simulink model "platoon_project"  (Simulink 8.9)
settings: Solver=FixedStepAuto  StartTime=0.0  StopTime=5  FixedStep=0.1  RelTol=1e-3  EnableMultiTasking=on
values from neighbouring files (symbols this model uses):
  tnet_table = [57.5127074443 119.897368421 182.282029398 223.675296349 261.549751738 274.206057597 279.305263158 283.689473684 288.073684211 292.467532318 296.875779086 301.284025854 ... (400 elements, 20x20)]    [enginemap.mat]    (also in genmap.m = griddata(map_ford(:,1), map_ford(:,4), map_ford(:,2), we_tab)
  we_max = 471.2    [enginemap.mat]    (also in genmap.m = max(map_ford(:,1)))
  we_min = 57.6    [enginemap.mat]    (also in genmap.m = min(map_ford(:,1)))
undefined symbols (not defined in the file or in its folder): c_aero, delay_brake, F_roll, h, I_e, I_wheel, KB, mass, max_throttle, max_throttle_rate, min_throttle, mu_B, mu_C, mu_D, mu_E, P_po, Rdrive, tau_brake, tau_throttle, throttle_o, w_wheel_o, we_o, x_dot_o
libraries: simulink x10
(part 3 of 3)

== system platoon_project/4th Vehicle/Wheel Dynamics/Left Front Wheel/Tire Model ==
  Wheel Speed : Inport
  Vehicle Speed : Inport  Port=2
  Constant : Constant  Value=0.01
  Constant1 : Constant  Value=0.01
  Fcn : Fcn  Expr=mu_D*sin(mu_C*atan(mu_B*u-mu_E*(mu_B*u-atan(mu_B*u))))
  Gain : Gain  SaturateOnIntegerOverflow=on  OutDataTypeStr=Inherit: Same as input  ParamDataTypeStr=Inherit: Same as input
  Product : Product  Inputs=/*  SaturateOnIntegerOverflow=on  RndMeth=Zero  InputSameDT=on  OutDataTypeStr=Inherit: Same as first input
  Product1 : Product  Inputs=*/  SaturateOnIntegerOverflow=on  RndMeth=Zero  InputSameDT=on  OutDataTypeStr=Inherit: Same as first input
  Sum1 : Sum  Inputs=+-  SaturateOnIntegerOverflow=on  InputSameDT=on  OutDataTypeStr=Inherit: Same as first input
  Switch : Switch  SaturateOnIntegerOverflow=on  InputSameDT=on
  Switch1 : Switch  Threshold=0.01  SaturateOnIntegerOverflow=on  InputSameDT=on
  Switch2 : Switch  Threshold=0.01  SaturateOnIntegerOverflow=on  InputSameDT=on
  wheel radius1 : Gain  Gain=h  SaturateOnIntegerOverflow=on  OutDataTypeStr=Inherit: Same as input  ParamDataTypeStr=Inherit: Same as input
  Tractive Force : Outport
  LF_slip : Outport  Port=2
  wires:
  wheel radius1/1 -> Sum1/1, Switch1/1, Switch1/2
  Sum1/1 -> Switch/2, Product/2, Product1/1
  Product/1 -> Switch/1
  Product1/1 -> Switch/3
  Switch/1 -> Gain/1, LF_slip/1  "slip"
  Wheel Speed/1 -> wheel radius1/1
  Fcn/1 -> Tractive Force/1
  Vehicle Speed/1 -> Sum1/2, Switch2/1, Switch2/2
  Gain/1 -> Fcn/1
  Constant/1 -> Switch1/3
  Switch1/1 -> Product/1
  Switch2/1 -> Product1/2
  Constant1/1 -> Switch2/3

== system platoon_project/4th Vehicle/Wheel Dynamics/Left Rear Wheel/Tire Model ==
  note: Magic Tire Formula
  note: rw-v
  note: Slip ratio
  note: divide by 0를 없애기 위해
      | Switch Block을 사용했다
  Wheel Speed : Inport
  Vehicle Speed : Inport  Port=2
  Constant : Constant  Value=0.01
  Constant1 : Constant  Value=0.01
  Fcn : Fcn  Expr=mu_D*sin(mu_C*atan(mu_B*u-mu_E*(mu_B*u-atan(mu_B*u))))
  Gain : Gain  SaturateOnIntegerOverflow=on  OutDataTypeStr=Inherit: Same as input  ParamDataTypeStr=Inherit: Same as input
  Product : Product  Inputs=/*  SaturateOnIntegerOverflow=on  RndMeth=Zero  InputSameDT=on  OutDataTypeStr=Inherit: Same as first input
  Product1 : Product  Inputs=*/  SaturateOnIntegerOverflow=on  RndMeth=Zero  InputSameDT=on  OutDataTypeStr=Inherit: Same as first input
  Sum1 : Sum  Inputs=+-  SaturateOnIntegerOverflow=on  InputSameDT=on  OutDataTypeStr=Inherit: Same as first input
  Switch : Switch  SaturateOnIntegerOverflow=on  InputSameDT=on
  Switch1 : Switch  Threshold=0.01  SaturateOnIntegerOverflow=on  InputSameDT=on
  Switch2 : Switch  Threshold=0.01  SaturateOnIntegerOverflow=on  InputSameDT=on
  wheel radius1 : Gain  Gain=h  SaturateOnIntegerOverflow=on  OutDataTypeStr=Inherit: Same as input  ParamDataTypeStr=Inherit: Same as input
  Tractive Force : Outport
  LR_slip : Outport  Port=2
  wires:
  wheel radius1/1 -> Sum1/1, Switch1/1, Switch1/2
  Sum1/1 -> Switch/2, Product/2, Product1/1
  Product/1 -> Switch/1
  Product1/1 -> Switch/3
  Switch/1 -> Gain/1, LR_slip/1  "slip"
  Wheel Speed/1 -> wheel radius1/1
  Fcn/1 -> Tractive Force/1
  Vehicle Speed/1 -> Sum1/2, Switch2/1, Switch2/2
  Gain/1 -> Fcn/1
  Constant/1 -> Switch1/3
  Switch1/1 -> Product/1
  Switch2/1 -> Product1/2
  Constant1/1 -> Switch2/3

== system platoon_project/4th Vehicle/Wheel Dynamics/Right Front Wheel/Tire Model ==
  note: rw-v
  note: Magic Tire Formula
  note: Slip ratio
  note: divide by 0를 없애기 위해
      | Switch Block을 사용했다
  Wheel Speed : Inport
  Vehicle Speed : Inport  Port=2
  Constant : Constant  Value=0.01
  Constant1 : Constant  Value=0.01
  Fcn : Fcn  Expr=mu_D*sin(mu_C*atan(mu_B*u-mu_E*(mu_B*u-atan(mu_B*u))))
  Gain : Gain  SaturateOnIntegerOverflow=on  OutDataTypeStr=Inherit: Same as input  ParamDataTypeStr=Inherit: Same as input
  Product : Product  Inputs=/*  SaturateOnIntegerOverflow=on  RndMeth=Zero  InputSameDT=on  OutDataTypeStr=Inherit: Same as first input
  Product1 : Product  Inputs=*/  SaturateOnIntegerOverflow=on  RndMeth=Zero  InputSameDT=on  OutDataTypeStr=Inherit: Same as first input
  Sum1 : Sum  Inputs=+-  SaturateOnIntegerOverflow=on  InputSameDT=on  OutDataTypeStr=Inherit: Same as first input
  Switch : Switch  SaturateOnIntegerOverflow=on  InputSameDT=on
  Switch1 : Switch  Threshold=0.01  SaturateOnIntegerOverflow=on  InputSameDT=on
  Switch2 : Switch  Threshold=0.01  SaturateOnIntegerOverflow=on  InputSameDT=on
  wheel radius1 : Gain  Gain=h  SaturateOnIntegerOverflow=on  OutDataTypeStr=Inherit: Same as input  ParamDataTypeStr=Inherit: Same as input
  Tractive Force : Outport
  RF_slip : Outport  Port=2
  wires:
  wheel radius1/1 -> Sum1/1, Switch1/1, Switch1/2
  Sum1/1 -> Switch/2, Product/2, Product1/1
  Product/1 -> Switch/1
  Product1/1 -> Switch/3
  Switch/1 -> Gain/1, RF_slip/1  "slip"
  Wheel Speed/1 -> wheel radius1/1
  Fcn/1 -> Tractive Force/1
  Vehicle Speed/1 -> Sum1/2, Switch2/1, Switch2/2
  Gain/1 -> Fcn/1
  Constant/1 -> Switch1/3
  Switch1/1 -> Product/1
  Switch2/1 -> Product1/2
  Constant1/1 -> Switch2/3

== system platoon_project/4th Vehicle/Wheel Dynamics/Right Rear Wheel/Tire Model ==
  Wheel Speed : Inport
  Vehicle Speed : Inport  Port=2
  Constant : Constant  Value=0.01
  Constant1 : Constant  Value=0.01
  Fcn : Fcn  Expr=mu_D*sin(mu_C*atan(mu_B*u-mu_E*(mu_B*u-atan(mu_B*u))))
  Gain : Gain  SaturateOnIntegerOverflow=on  OutDataTypeStr=Inherit: Same as input  ParamDataTypeStr=Inherit: Same as input
  Product : Product  Inputs=/*  SaturateOnIntegerOverflow=on  RndMeth=Zero  InputSameDT=on  OutDataTypeStr=Inherit: Same as first input
  Product1 : Product  Inputs=*/  SaturateOnIntegerOverflow=on  RndMeth=Zero  InputSameDT=on  OutDataTypeStr=Inherit: Same as first input
  Sum1 : Sum  Inputs=+-  SaturateOnIntegerOverflow=on  InputSameDT=on  OutDataTypeStr=Inherit: Same as first input
  Switch : Switch  SaturateOnIntegerOverflow=on  InputSameDT=on
  Switch1 : Switch  Threshold=0.01  SaturateOnIntegerOverflow=on  InputSameDT=on
  Switch2 : Switch  Threshold=0.01  SaturateOnIntegerOverflow=on  InputSameDT=on
  wheel radius1 : Gain  Gain=h  SaturateOnIntegerOverflow=on  OutDataTypeStr=Inherit: Same as input  ParamDataTypeStr=Inherit: Same as input
  Tractive Force : Outport
  RR_slip : Outport  Port=2
  wires:
  wheel radius1/1 -> Sum1/1, Switch1/1, Switch1/2
  Sum1/1 -> Switch/2, Product/2, Product1/1
  Product/1 -> Switch/1
  Product1/1 -> Switch/3
  Switch/1 -> Gain/1, RR_slip/1  "slip"
  Wheel Speed/1 -> wheel radius1/1
  Fcn/1 -> Tractive Force/1
  Vehicle Speed/1 -> Sum1/2, Switch2/1, Switch2/2
  Gain/1 -> Fcn/1
  Constant/1 -> Switch1/3
  Switch1/1 -> Product/1
  Switch2/1 -> Product1/2
  Constant1/1 -> Switch2/3

== system platoon_project/Lead Vehicle/Wheel Dynamics/Left Front Wheel/Tire Model ==
  Wheel Speed : Inport
  Vehicle Speed : Inport  Port=2
  Constant : Constant  Value=0.01
  Constant1 : Constant  Value=0.01
  Fcn : Fcn  Expr=mu_D*sin(mu_C*atan(mu_B*u-mu_E*(mu_B*u-atan(mu_B*u))))
  Gain : Gain  SaturateOnIntegerOverflow=on  OutDataTypeStr=Inherit: Same as input  ParamDataTypeStr=Inherit: Same as input
  Product : Product  Inputs=/*  SaturateOnIntegerOverflow=on  RndMeth=Zero  InputSameDT=on  OutDataTypeStr=Inherit: Same as first input
  Product1 : Product  Inputs=*/  SaturateOnIntegerOverflow=on  RndMeth=Zero  InputSameDT=on  OutDataTypeStr=Inherit: Same as first input
  Sum1 : Sum  Inputs=+-  SaturateOnIntegerOverflow=on  InputSameDT=on  OutDataTypeStr=Inherit: Same as first input
  Switch : Switch  SaturateOnIntegerOverflow=on  InputSameDT=on
  Switch1 : Switch  Threshold=0.01  SaturateOnIntegerOverflow=on  InputSameDT=on
  Switch2 : Switch  Threshold=0.01  SaturateOnIntegerOverflow=on  InputSameDT=on
  wheel radius1 : Gain  Gain=h  SaturateOnIntegerOverflow=on  OutDataTypeStr=Inherit: Same as input  ParamDataTypeStr=Inherit: Same as input
  Tractive Force : Outport
  LF_slip : Outport  Port=2
  wires:
  wheel radius1/1 -> Sum1/1, Switch1/1, Switch1/2
  Sum1/1 -> Switch/2, Product/2, Product1/1
  Product/1 -> Switch/1
  Product1/1 -> Switch/3
  Switch/1 -> Gain/1, LF_slip/1  "slip"
  Wheel Speed/1 -> wheel radius1/1
  Fcn/1 -> Tractive Force/1
  Vehicle Speed/1 -> Sum1/2, Switch2/1, Switch2/2
  Gain/1 -> Fcn/1
  Constant/1 -> Switch1/3
  Switch1/1 -> Product/1
  Switch2/1 -> Product1/2
  Constant1/1 -> Switch2/3

== system platoon_project/Lead Vehicle/Wheel Dynamics/Left Rear Wheel/Tire Model ==
  note: Magic Tire Formula
  note: rw-v
  note: Slip ratio
  note: divide by 0를 없애기 위해
      | Switch Block을 사용했다
  Wheel Speed : Inport
  Vehicle Speed : Inport  Port=2
  Constant : Constant  Value=0.01
  Constant1 : Constant  Value=0.01
  Fcn : Fcn  Expr=mu_D*sin(mu_C*atan(mu_B*u-mu_E*(mu_B*u-atan(mu_B*u))))
  Gain : Gain  SaturateOnIntegerOverflow=on  OutDataTypeStr=Inherit: Same as input  ParamDataTypeStr=Inherit: Same as input
  Product : Product  Inputs=/*  SaturateOnIntegerOverflow=on  RndMeth=Zero  InputSameDT=on  OutDataTypeStr=Inherit: Same as first input
  Product1 : Product  Inputs=*/  SaturateOnIntegerOverflow=on  RndMeth=Zero  InputSameDT=on  OutDataTypeStr=Inherit: Same as first input
  Sum1 : Sum  Inputs=+-  SaturateOnIntegerOverflow=on  InputSameDT=on  OutDataTypeStr=Inherit: Same as first input
  Switch : Switch  SaturateOnIntegerOverflow=on  InputSameDT=on
  Switch1 : Switch  Threshold=0.01  SaturateOnIntegerOverflow=on  InputSameDT=on
  Switch2 : Switch  Threshold=0.01  SaturateOnIntegerOverflow=on  InputSameDT=on
  wheel radius1 : Gain  Gain=h  SaturateOnIntegerOverflow=on  OutDataTypeStr=Inherit: Same as input  ParamDataTypeStr=Inherit: Same as input
  Tractive Force : Outport
  LR_slip : Outport  Port=2
  wires:
  wheel radius1/1 -> Sum1/1, Switch1/1, Switch1/2
  Sum1/1 -> Switch/2, Product/2, Product1/1
  Product/1 -> Switch/1
  Product1/1 -> Switch/3
  Switch/1 -> Gain/1, LR_slip/1  "slip"
  Wheel Speed/1 -> wheel radius1/1
  Fcn/1 -> Tractive Force/1
  Vehicle Speed/1 -> Sum1/2, Switch2/1, Switch2/2
  Gain/1 -> Fcn/1
  Constant/1 -> Switch1/3
  Switch1/1 -> Product/1
  Switch2/1 -> Product1/2
  Constant1/1 -> Switch2/3

== system platoon_project/Lead Vehicle/Wheel Dynamics/Right Front Wheel/Tire Model ==
  note: rw-v
  note: Magic Tire Formula
  note: Slip ratio
  note: divide by 0를 없애기 위해
      | Switch Block을 사용했다
  Wheel Speed : Inport
  Vehicle Speed : Inport  Port=2
  Constant : Constant  Value=0.01
  Constant1 : Constant  Value=0.01
  Fcn : Fcn  Expr=mu_D*sin(mu_C*atan(mu_B*u-mu_E*(mu_B*u-atan(mu_B*u))))
  Gain : Gain  SaturateOnIntegerOverflow=on  OutDataTypeStr=Inherit: Same as input  ParamDataTypeStr=Inherit: Same as input
  Product : Product  Inputs=/*  SaturateOnIntegerOverflow=on  RndMeth=Zero  InputSameDT=on  OutDataTypeStr=Inherit: Same as first input
  Product1 : Product  Inputs=*/  SaturateOnIntegerOverflow=on  RndMeth=Zero  InputSameDT=on  OutDataTypeStr=Inherit: Same as first input
  Sum1 : Sum  Inputs=+-  SaturateOnIntegerOverflow=on  InputSameDT=on  OutDataTypeStr=Inherit: Same as first input
  Switch : Switch  SaturateOnIntegerOverflow=on  InputSameDT=on
  Switch1 : Switch  Threshold=0.01  SaturateOnIntegerOverflow=on  InputSameDT=on
  Switch2 : Switch  Threshold=0.01  SaturateOnIntegerOverflow=on  InputSameDT=on
  wheel radius1 : Gain  Gain=h  SaturateOnIntegerOverflow=on  OutDataTypeStr=Inherit: Same as input  ParamDataTypeStr=Inherit: Same as input
  Tractive Force : Outport
  RF_slip : Outport  Port=2
  wires:
  wheel radius1/1 -> Sum1/1, Switch1/1, Switch1/2
  Sum1/1 -> Switch/2, Product/2, Product1/1
  Product/1 -> Switch/1
  Product1/1 -> Switch/3
  Switch/1 -> Gain/1, RF_slip/1  "slip"
  Wheel Speed/1 -> wheel radius1/1
  Fcn/1 -> Tractive Force/1
  Vehicle Speed/1 -> Sum1/2, Switch2/1, Switch2/2
  Gain/1 -> Fcn/1
  Constant/1 -> Switch1/3
  Switch1/1 -> Product/1
  Switch2/1 -> Product1/2
  Constant1/1 -> Switch2/3

== system platoon_project/Lead Vehicle/Wheel Dynamics/Right Rear Wheel/Tire Model ==
  Wheel Speed : Inport
  Vehicle Speed : Inport  Port=2
  Constant : Constant  Value=0.01
  Constant1 : Constant  Value=0.01
  Fcn : Fcn  Expr=mu_D*sin(mu_C*atan(mu_B*u-mu_E*(mu_B*u-atan(mu_B*u))))
  Gain : Gain  SaturateOnIntegerOverflow=on  OutDataTypeStr=Inherit: Same as input  ParamDataTypeStr=Inherit: Same as input
  Product : Product  Inputs=/*  SaturateOnIntegerOverflow=on  RndMeth=Zero  InputSameDT=on  OutDataTypeStr=Inherit: Same as first input
  Product1 : Product  Inputs=*/  SaturateOnIntegerOverflow=on  RndMeth=Zero  InputSameDT=on  OutDataTypeStr=Inherit: Same as first input
  Sum1 : Sum  Inputs=+-  SaturateOnIntegerOverflow=on  InputSameDT=on  OutDataTypeStr=Inherit: Same as first input
  Switch : Switch  SaturateOnIntegerOverflow=on  InputSameDT=on
  Switch1 : Switch  Threshold=0.01  SaturateOnIntegerOverflow=on  InputSameDT=on
  Switch2 : Switch  Threshold=0.01  SaturateOnIntegerOverflow=on  InputSameDT=on
  wheel radius1 : Gain  Gain=h  SaturateOnIntegerOverflow=on  OutDataTypeStr=Inherit: Same as input  ParamDataTypeStr=Inherit: Same as input
  Tractive Force : Outport
  RR_slip : Outport  Port=2
  wires:
  wheel radius1/1 -> Sum1/1, Switch1/1, Switch1/2
  Sum1/1 -> Switch/2, Product/2, Product1/1
  Product/1 -> Switch/1
  Product1/1 -> Switch/3
  Switch/1 -> Gain/1, RR_slip/1  "slip"
  Wheel Speed/1 -> wheel radius1/1
  Fcn/1 -> Tractive Force/1
  Vehicle Speed/1 -> Sum1/2, Switch2/1, Switch2/2
  Gain/1 -> Fcn/1
  Constant/1 -> Switch1/3
  Switch1/1 -> Product/1
  Switch2/1 -> Product1/2
  Constant1/1 -> Switch2/3

== matlab function                ACC Based On DIstance             ==
  data: frontSpeed input double; rearSpeed input double; Throttle_Angle_err output double; distance input double; Pmc_err output double
function [Throttle_Angle_err,Pmc_err] = acc(frontSpeed,rearSpeed, distance)

timeC=0.1;   % dt [s]
acc_C = 10.19; % 최대 브레이크 감가속도 [m/s^2]
minSpeed = 10;    % 최소 속도 [m/s]
des_distance=10;  % 목표 거리 [m]

persistent setSpeed;

if isempty(setSpeed)
    setSpeed= 0;
end

% 등가속도 법칙에서 s = (vf^2 - vr^2) / 2a를 사용해서 rear vehicle이 dt동안 이동할 거리 구한다
% 너무 가까워지면 브레이크를 밟아야하므로 중요하다
deltaX = ((frontSpeed*frontSpeed)-(rearSpeed*rearSpeed))/(2*(-acc_C));

if deltaX < 0
    Throttle_Angle_err =  0;
    Pmc_err =  1; 
    return 
end

if(distance<=(des_distance + (deltaX)))
    % 실제거리가 des_distance + deltaX 구간에 있는 경우
    if(distance <= deltaX + des_distance) && (distance  >= des_distance)
        tmpSpeed1 = sqrt((rearSpeed * rearSpeed) + (2*(-acc_C)*abs((deltaX + des_distance)-distance)));
        setSpeed = max(frontSpeed,tmpSpeed1);      % stops the reduction at front_speed.
        
    % 실제거리가 des_distance보다 가까이 있는 경우
    elseif(distance < des_distance)
        tmpSpeed2 = sqrt((rearSpeed * rearSpeed) + (2*(-acc_C)*abs(des_distance-distance)));
        setSpeed = max(minSpeed,tmpSpeed2);
    end

% 실제거리가 des_distane보다 멀리 있는 경우
elseif (distance>(des_distance + (deltaX)))
    setSpeed = rearSpeed + (acc_C * timeC);   % v = u + at
end

% 실제속도와 계산된 다음 속도의 차이를 반환합니다
diffSpeed = setSpeed - rearSpeed;

if diffSpeed > 0
    Throttle_Angle_err =  1;
    Pmc_err = 0;
else 
    Throttle_Angle_err =  0;
    Pmc_err =  1; 
end


end

== matlab function                ACC Based On DIstance            ==
  data: frontSpeed input double; rearSpeed input double; Throttle_Angle_err output double; distance input double; Pmc_err output double
function [Throttle_Angle_err,Pmc_err] = acc(frontSpeed,rearSpeed, distance)

timeC=0.1;   % dt [s]
acc_C = 10.19; % 최대 브레이크 감가속도 [m/s^2]
minSpeed = 10;    % 최소 속도 [m/s]
des_distance=10;  % 목표 거리 [m]

persistent setSpeed;

if isempty(setSpeed)
    setSpeed= 0;
end

% 등가속도 법칙에서 s = (vf^2 - vr^2) / 2a를 사용해서 rear vehicle이 dt동안 이동할 거리 구한다
% 너무 가까워지면 브레이크를 밟아야하므로 중요하다
deltaX = ((frontSpeed*frontSpeed)-(rearSpeed*rearSpeed))/(2*(-acc_C));

if deltaX < 0
    Throttle_Angle_err =  0;
    Pmc_err =  1; 
    return 
end

if(distance<=(des_distance + (deltaX)))
    % 실제거리가 des_distance + deltaX 구간에 있는 경우
    if(distance <= deltaX + des_distance) && (distance  >= des_distance)
        tmpSpeed1 = sqrt((rearSpeed * rearSpeed) + (2*(-acc_C)*abs((deltaX + des_distance)-distance)));
        setSpeed = max(frontSpeed,tmpSpeed1);      % stops the reduction at front_speed.
        
    % 실제거리가 des_distance보다 가까이 있는 경우
    elseif(distance < des_distance)
        tmpSpeed2 = sqrt((rearSpeed * rearSpeed) + (2*(-acc_C)*abs(des_distance-distance)));
        setSpeed = max(minSpeed,tmpSpeed2);
    end

% 실제거리가 des_distane보다 멀리 있는 경우
elseif (distance>(des_distance + (deltaX)))
    setSpeed = rearSpeed + (acc_C * timeC);   % v = u + at
end

% 실제속도와 계산된 다음 속도의 차이를 반환합니다
diffSpeed = setSpeed - rearSpeed;

if diffSpeed > 0
    Throttle_Angle_err =  1;
    Pmc_err = 0;
else 
    Throttle_Angle_err =  0;
    Pmc_err =  1; 
end


end

== matlab function                 ACC Based On DIstance            ==
  data: frontSpeed input double; rearSpeed input double; Throttle_Angle_err output double; distance input double; Pmc_err output double
function [Throttle_Angle_err,Pmc_err] = acc(frontSpeed,rearSpeed, distance)

timeC=0.1;   % dt [s]
acc_C = 10.19; % 최대 브레이크 감가속도 [m/s^2]
minSpeed = 10;    % 최소 속도 [m/s]
des_distance=10;  % 목표 거리 [m]

persistent setSpeed;

if isempty(setSpeed)
    setSpeed= 0;
end

% 등가속도 법칙에서 s = (vf^2 - vr^2) / 2a를 사용해서 rear vehicle이 dt동안 이동할 거리 구한다
% 너무 가까워지면 브레이크를 밟아야하므로 중요하다
deltaX = ((frontSpeed*frontSpeed)-(rearSpeed*rearSpeed))/(2*(-acc_C));

if deltaX < 0
    Throttle_Angle_err =  0;
    Pmc_err =  1; 
    return 
end

if(distance<=(des_distance + (deltaX)))
    % 실제거리가 des_distance + deltaX 구간에 있는 경우
    if(distance <= deltaX + des_distance) && (distance  >= des_distance)
        tmpSpeed1 = sqrt((rearSpeed * rearSpeed) + (2*(-acc_C)*abs((deltaX + des_distance)-distance)));
        setSpeed = max(frontSpeed,tmpSpeed1);      % stops the reduction at front_speed.
        
    % 실제거리가 des_distance보다 가까이 있는 경우
    elseif(distance < des_distance)
        tmpSpeed2 = sqrt((rearSpeed * rearSpeed) + (2*(-acc_C)*abs(des_distance-distance)));
        setSpeed = max(minSpeed,tmpSpeed2);
    end

% 실제거리가 des_distane보다 멀리 있는 경우
elseif (distance>(des_distance + (deltaX)))
    setSpeed = rearSpeed + (acc_C * timeC);   % v = u + at
end

% 실제속도와 계산된 다음 속도의 차이를 반환합니다
diffSpeed = setSpeed - rearSpeed;

if diffSpeed > 0
    Throttle_Angle_err =  1;
    Pmc_err = 0;
else 
    Throttle_Angle_err =  0;
    Pmc_err =  1; 
end


end

== matlab function                ACC Based On DIstance              ==
  data: frontSpeed input double; rearSpeed input double; Throttle_Angle_err output double; distance input double; Pmc_err output double
function [Throttle_Angle_err,Pmc_err] = acc(frontSpeed,rearSpeed, distance)

timeC=0.1;   % dt [s]
acc_C = 10.19; % 최대 브레이크 감가속도 [m/s^2]
minSpeed = 10;    % 최소 속도 [m/s]
des_distance=10;  % 목표 거리 [m]

persistent setSpeed;

if isempty(setSpeed)
    setSpeed= 0;
end

% 등가속도 법칙에서 s = (vf^2 - vr^2) / 2a를 사용해서 rear vehicle이 dt동안 이동할 거리 구한다
% 너무 가까워지면 브레이크를 밟아야하므로 중요하다
deltaX = ((frontSpeed*frontSpeed)-(rearSpeed*rearSpeed))/(2*(-acc_C));

if deltaX < 0
    Throttle_Angle_err =  0;
    Pmc_err =  1; 
    return 
end

if(distance<=(des_distance + (deltaX)))
    % 실제거리가 des_distance + deltaX 구간에 있는 경우
    if(distance <= deltaX + des_distance) && (distance  >= des_distance)
        tmpSpeed1 = sqrt((rearSpeed * rearSpeed) + (2*(-acc_C)*abs((deltaX + des_distance)-distance)));
        setSpeed = max(frontSpeed,tmpSpeed1);      % stops the reduction at front_speed.
        
    % 실제거리가 des_distance보다 가까이 있는 경우
    elseif(distance < des_distance)
        tmpSpeed2 = sqrt((rearSpeed * rearSpeed) + (2*(-acc_C)*abs(des_distance-distance)));
        setSpeed = max(minSpeed,tmpSpeed2);
    end

% 실제거리가 des_distane보다 멀리 있는 경우
elseif (distance>(des_distance + (deltaX)))
    setSpeed = rearSpeed + (acc_C * timeC);   % v = u + at
end

% 실제속도와 계산된 다음 속도의 차이를 반환합니다
diffSpeed = setSpeed - rearSpeed;

if diffSpeed > 0
    Throttle_Angle_err =  1;
    Pmc_err = 0;
else 
    Throttle_Angle_err =  0;
    Pmc_err =  1; 
end


end
